simulink model "scheme2"  (R2014a)
settings: Solver=ode45  StartTime=0.0  StopTime=10.0  RelTol=1e-3
libraries: simulink x1
settings Model: Creator=Valentin  LastModifiedBy=Valentin

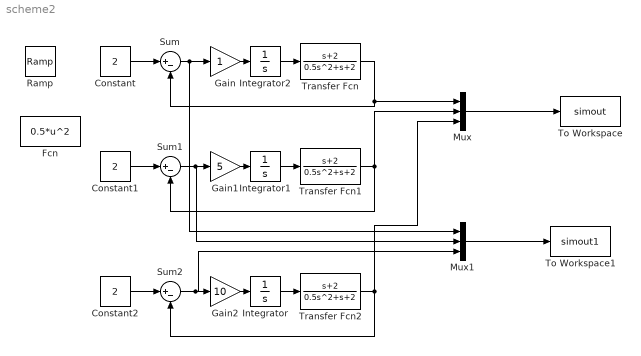
== system scheme2 ==
  Constant : Constant  Value=2
  Constant1 : Constant  Value=2
  Constant2 : Constant  Value=2
  Fcn : Fcn  Expr=0.5*u^2
  Gain : Gain
  Gain1 : Gain  Gain=5
  Gain2 : Gain  Gain=10
  Integrator : Integrator
  Integrator1 : Integrator
  Integrator2 : Integrator
  Mux : Mux  Inputs=3
  Mux1 : Mux  Inputs=3
  Ramp : simulink/Sources/Ramp  slope=2  start=0  X0=0
  Sum : Sum  Inputs=|+-
  Sum1 : Sum  Inputs=|+-
  Sum2 : Sum  Inputs=|+-
  To Workspace : ToWorkspace  VariableName=simout  SaveFormat=Timeseries  SampleTime=-1
  To Workspace1 : ToWorkspace  VariableName=simout1  SaveFormat=Timeseries  SampleTime=-1
  Transfer Fcn : TransferFcn  Numerator=[1 2]  Denominator=[0.5 1 2]
  Transfer Fcn1 : TransferFcn  Numerator=[1 2]  Denominator=[0.5 1 2]
  Transfer Fcn2 : TransferFcn  Numerator=[1 2]  Denominator=[0.5 1 2]
  wires:
  Transfer Fcn/1 -> Mux/1, Sum/2
  Constant/1 -> Sum/1
  Sum/1 -> Mux1/1, Gain/1
  Transfer Fcn1/1 -> Sum1/2, Mux/2
  Constant1/1 -> Sum1/1
  Sum1/1 -> Mux1/2, Gain1/1
  Transfer Fcn2/1 -> Sum2/2, Mux/3
  Constant2/1 -> Sum2/1
  Sum2/1 -> Mux1/3, Gain2/1
  Mux/1 -> To Workspace/1
  Mux1/1 -> To Workspace1/1
  Gain/1 -> Integrator2/1
  Integrator2/1 -> Transfer Fcn/1
  Gain1/1 -> Integrator1/1
  Integrator1/1 -> Transfer Fcn1/1
  Gain2/1 -> Integrator/1
  Integrator/1 -> Transfer Fcn2/1
